simulink model "task1_diag"  (R2024a)
settings: Solver=VariableStepAuto  StartTime=0.0  StopTime=10.0  RelTol=1e-3
settings Model: Creator=sizgr  LastModifiedBy=sizgr

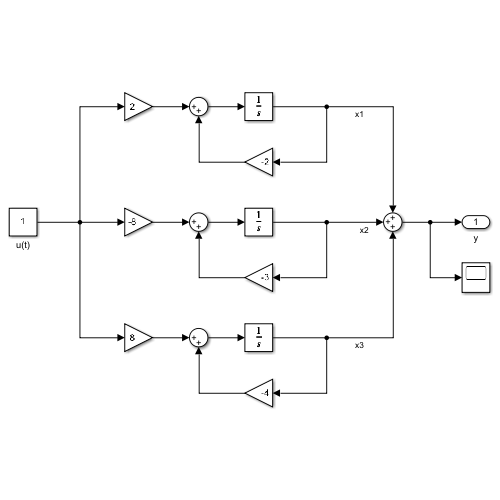
[thumbnail: Simulink's stored preview of the top-level diagram]
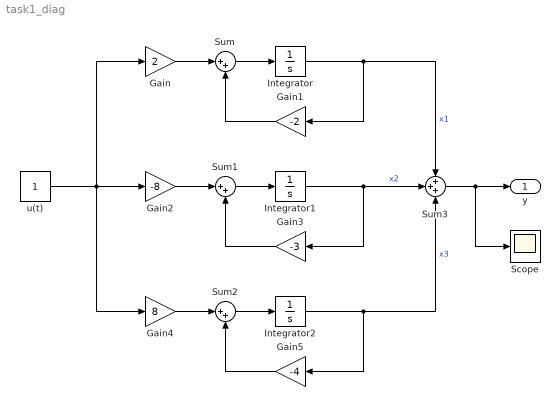
== system task1_diag ==
  Gain : Gain  Gain=2
  Gain1 : Gain  Gain=-2
  Gain2 : Gain  Gain=-8
  Gain3 : Gain  Gain=-3
  Gain4 : Gain  Gain=8
  Gain5 : Gain  Gain=-4
  Integrator : Integrator
  Integrator1 : Integrator
  Integrator2 : Integrator
  Scope : Scope
  Sum : Sum  Inputs=|++
  Sum1 : Sum  Inputs=|++
  Sum2 : Sum  Inputs=|++
  Sum3 : Sum  Inputs=+++
  u(t) : Constant
  y : Outport
  wires:
  Gain/1 -> Sum/1
  Sum/1 -> Integrator/1
  Gain1/1 -> Sum/2
  Integrator/1 -> Sum3/1, Gain1/1  "x1"
  Integrator1/1 -> Sum3/2, Gain3/1  "x2"
  Gain3/1 -> Sum1/2
  Sum1/1 -> Integrator1/1
  Gain2/1 -> Sum1/1
  Integrator2/1 -> Sum3/3, Gain5/1  "x3"
  Gain5/1 -> Sum2/2
  Sum2/1 -> Integrator2/1
  Gain4/1 -> Sum2/1
  u(t)/1 -> Gain4/1, Gain/1, Gain2/1
  Sum3/1 -> Scope/1, y/1
